simulink library "lib_FaultDetection"  (R2017a)
settings: Solver=VariableStepAuto  StartTime=0.0  StopTime=10.0  RelTol=1e-3
undefined symbols (not defined in the file): cal, ENGTRQ_MSMCH_Degraded_CP, ENGTRQ_MSMCH_ErrCritical_CP, ENGTRQ_MSMCH_LimpHome_CP
libraries: simulink x57, Diagnostic x4, lib_SystemDiag x1
(part 2 of 3)

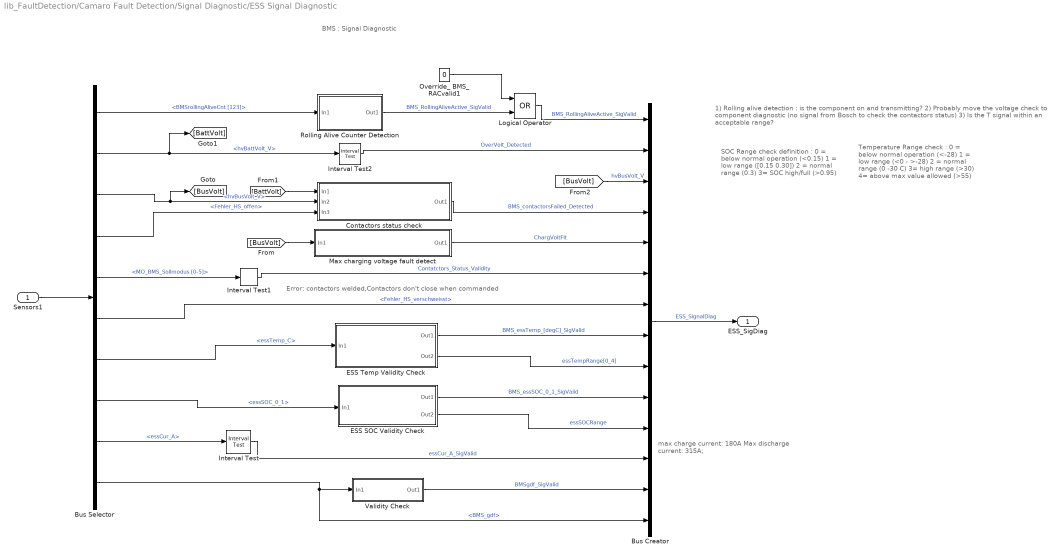
== system lib_FaultDetection/Camaro Fault Detection/Signal Diagnostic/ESS Signal Diagnostic ==
  note: BMS : Signal Diagnostic
  note: 1) Rolling alive detection : is the component on and transmitting?
      | 2) Probably move the voltage check to component diagnostic (no signal from Bosch to check the contactors status)
      | 3) Is  the T signal within an acceptable range?
  note: SOC Range check definition :
      | 0 = below normal operation (<0.15)
      | 1 = low range ([0.15 0.30])
      | 2 = normal range (0.3)
      | 3= SOC high/full (>0.95)
  note: Temperature Range check :
      | 0 = below normal operation (<-28)
      | 1 = low range (<0 - >-28)
      | 2 = normal range (0 -30 C)
      | 3= high range (>30)
      | 4= above max value allowed (>55)
  note: Error: contactors welded,Contactors don't close when commanded
  note: max charge current: 180A
      | Max discharge current: 315A;
  Sensors1 : Inport
  Bus Creator : BusCreator  Inputs=14
  Bus Selector : BusSelector  OutputSignals=BMS_Conv.BMSrollingAliveCnt [123],BMS_Conv.hvBattVolt_V,BMS_Conv.hvBusVolt_V,BMS_Conv.Fehler_HS_offen,BMS_Conv.MO_BMS_Sollmodus [0-5],BMS_Conv.Fehler_HS_verschweisst,BMS_Conv.essTemp_C,BMS_Conv.essSOC_0_1,BMS_Conv.essCur_A,BMS_Conv.BMS_gdf
  Contactors status check : Subsystem
  ESS SOC Validity Check : Subsystem
  ESS Temp Validity Check : Subsystem
  Interval Test : simulink/Logic and Bit Operations/Interval Test  IntervalClosedRight=on  uplimit=180  IntervalClosedLeft=on  lowlimit=-315  OutDataTypeStr=boolean
  Interval Test1 : simulink/Logic and Bit Operations/Interval Test  IntervalClosedRight=on  uplimit=7  IntervalClosedLeft=on  lowlimit=0  OutDataTypeStr=boolean
  Interval Test2 : simulink/Logic and Bit Operations/Interval Test  IntervalClosedRight=on  uplimit=430  IntervalClosedLeft=on  lowlimit=291  OutDataTypeStr=boolean
  Logical Operator : Logic  Operator=OR  AllPortsSameDT=off  OutDataTypeStr=boolean
  Max charging voltage fault detect : Subsystem
  Override_ BMS_RACvalid1 : Constant  Value=0
  Rolling Alive Counter Detection : Subsystem
  Validity Check : Subsystem
  ESS_SigDiag : Outport
  wires:
  Override_ BMS_RACvalid1/1 -> Logical Operator/1
  Rolling Alive Counter Detection/1(Out1) -> Logical Operator/2  "BMS_RollingAliveActive_SigValid"
  [BusVolt] -> Bus Creator/3  "hvBusVolt_V"
  Max charging voltage fault detect/1(Out1) -> Bus Creator/5  "ChargVoltFlt"
  [BusVolt] -> Max charging voltage fault detect/1(In1)
  [BattVolt] -> Contactors status check/1(In1)
  Interval Test2/1 -> Bus Creator/2  "OverVolt_Detected"
  Interval Test1/1 -> Bus Creator/6  "Contatctors_Status_Validity"
  Bus Selector/5 -> Interval Test1/1  "<MO_BMS_Sollmodus [0-5]>"
  Bus Selector/6 -> Bus Creator/7  "<Fehler_HS_verschweisst>"
  Contactors status check/1(Out1) -> Bus Creator/4  "BMS_contactorsFailed_Detected"
  Bus Selector/4 -> Contactors status check/3(In3)  "<Fehler_HS_offen>"
  Bus Selector/3 -> [BusVolt], Contactors status check/2(In2)  "<hvBusVolt_V>"
  ESS Temp Validity Check/2(Out2) -> Bus Creator/9  "essTempRange[0_4]"
  ESS Temp Validity Check/1(Out1) -> Bus Creator/8  "BMS_essTemp_[degC]_SigValid"
  Bus Selector/7 -> ESS Temp Validity Check/1(In1)  "<essTemp_C>"
  ESS SOC Validity Check/2(Out2) -> Bus Creator/11  "essSOCRange"
  ESS SOC Validity Check/1(Out1) -> Bus Creator/10  "BMS_essSOC_0_1_SigValid"
  Bus Selector/8 -> ESS SOC Validity Check/1(In1)  "<essSOC_0_1>"
  Validity Check/1(Out1) -> Bus Creator/13  "BMSgdf_SigValid"
  Bus Selector/10 -> Validity Check/1(In1), Bus Creator/14  "<BMS_gdf>"
  Interval Test/1 -> Bus Creator/12  "essCur_A_SigValid"
  Bus Selector/9 -> Interval Test/1  "<essCur_A>"
  Bus Creator/1 -> ESS_SigDiag/1  "ESS_SignalDiag"
  Bus Selector/2 -> [BattVolt], Interval Test2/1  "<hvBattVolt_V>"
  Logical Operator/1 -> Bus Creator/1  "BMS_RollingAliveActive_SigValid"
  Bus Selector/1 -> Rolling Alive Counter Detection/1(In1)  "<BMSrollingAliveCnt [123]>"
  Sensors1/1 -> Bus Selector/1

== system lib_FaultDetection/Camaro Fault Detection/Signal Diagnostic/Engine Signal Diagnostic ==
  note: Engine_Temp:
      | Normal range: <100
      | above max:>120
      | Limited range: 100-120
  note: ECM : Signal Diagnostic
  Sensors1 : Inport
  Bus Creator : BusCreator  Inputs=9
  Bus Selector : BusSelector  OutputSignals=ECM_Conv.ECMrollingAliveCnt [123],ECM_Conv.ECMTrqCmd_Nm,ECM_Conv.EngActStdyStTorq_Nm,ECM_Conv.EngineSpeed_rpm,ECM_Conv.Engine_Temp[DegC],ECM_Conv.EngRunAtv
  Constant1 : Constant
  Eng Feedback Trq Range Valid? : simulink/Logic and Bit Operations/Interval Test  IntervalClosedRight=on  uplimit=233  IntervalClosedLeft=on  lowlimit=0  OutDataTypeStr=boolean
  Eng Trq Range Valid? : simulink/Logic and Bit Operations/Interval Test  IntervalClosedRight=on  uplimit=233  IntervalClosedLeft=on  lowlimit=0  OutDataTypeStr=boolean
  EngTempValidity_Check : Subsystem
  Engine Run Active Valid? : simulink/Logic and Bit Operations/Interval Test  IntervalClosedRight=on  uplimit=1  IntervalClosedLeft=on  lowlimit=0  OutDataTypeStr=boolean
  Engine Speed Range Valid? : simulink/Logic and Bit Operations/Interval Test  IntervalClosedRight=on  uplimit=6500  IntervalClosedLeft=on  lowlimit=0  OutDataTypeStr=boolean
  Engine_Temp[DegC] : Stateflow chart  TreatAsAtomicUnit=on
  Rolling Alive Counter Detection1 : Subsystem
  Engine_SigDiag : Outport
  wires:
  EngTempValidity_Check/1(Out1) -> Bus Creator/7  "Eng_TempValid"
  Engine_Temp[DegC]/1(EngTempRange) -> Bus Creator/8, EngTempValidity_Check/1(In1)  "Eng_TempRange[123]"
  Constant1/1 -> Engine_Temp[DegC]/1(clearFaults)
  Engine Run Active Valid?/1 -> Bus Creator/9  "EngRunAtValid"
  Bus Selector/6 -> Engine Run Active Valid?/1  "<EngRunAtv>"
  Bus Selector/5 -> Engine_Temp[DegC]/2(Engine_Temp_DegC)  "<Engine_Temp[DegC]>"
  Eng Feedback Trq Range Valid?/1 -> Bus Creator/4  "EngActStdyStTorq_SigValid"
  Bus Selector/3 -> Eng Feedback Trq Range Valid?/1, Bus Creator/5  "<EngActStdyStTorq_Nm>"
  Engine Speed Range Valid?/1 -> Bus Creator/6  "Engine_Speed_rpm_SigValid"
  Bus Selector/4 -> Engine Speed Range Valid?/1  "<EngineSpeed_rpm>"
  Bus Creator/1 -> Engine_SigDiag/1  "Engine_SignalDiag"
  Eng Trq Range Valid?/1 -> Bus Creator/3  "engTrqCmdRecvd_SigValid"
  Bus Selector/2 -> Eng Trq Range Valid?/1, Bus Creator/2  "<ECMTrqCmd_Nm>"
  Rolling Alive Counter Detection1/1(Out1) -> Bus Creator/1  "ECMRollingAliveActive"
  Bus Selector/1 -> Rolling Alive Counter Detection1/1(In1)  "<ECMrollingAliveCnt [123]>"
  Sensors1/1 -> Bus Selector/1

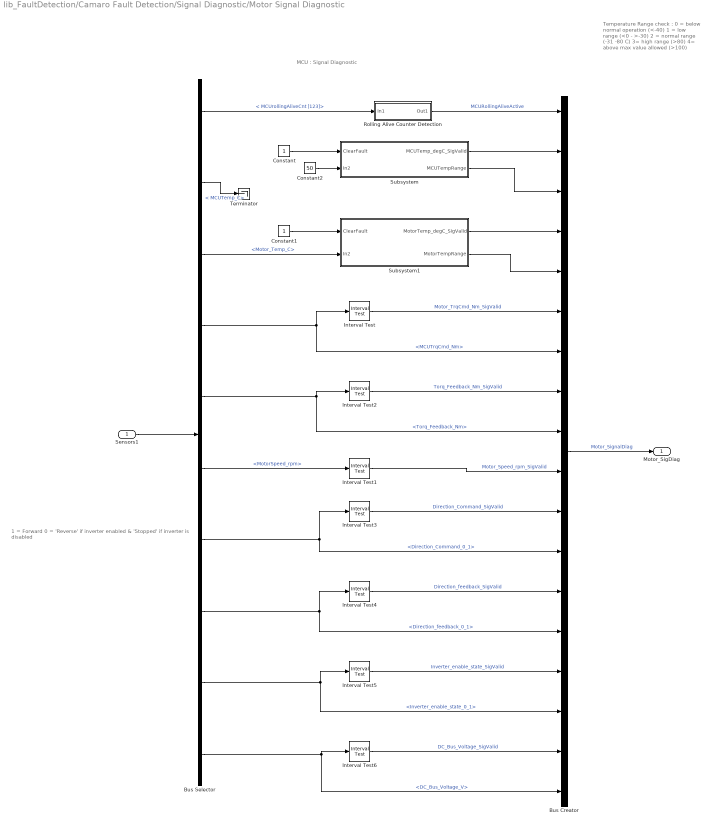
== system lib_FaultDetection/Camaro Fault Detection/Signal Diagnostic/Motor Signal Diagnostic ==
  note: 1 = Forward
      | 0 = 'Reverse' if inverter enabled  & 'Stopped' if inverter is disabled
  note: MCU : Signal Diagnostic
  note: Temperature Range check :
      | 0 = below normal operation (<-40)
      | 1 = low range (<0 - >-30)
      | 2 = normal range (-31 -80 C)
      | 3= high range (>80)
      | 4= above max value allowed (>100)
  Sensors1 : Inport
  Bus Creator : BusCreator  Inputs=18
  Bus Selector : BusSelector  OutputSignals=MCU_Conv.MCUrollingAliveCnt [123],MCU_Conv.MCUTemp_C,MCU_Conv.Motor_Temp_C,MCU_Conv.MCUTrqCmd_Nm,MCU_Conv.Torq_Feedback_Nm,MCU_Conv.MotorSpeed_rpm,MCU_Conv.Direction_Command_0_1,MCU_Conv.Direction_feedback_0_1,MCU_Conv.Inverter_enable_state_0_1,MCU_Conv.DC_Bus_Voltage_V
  Constant : Constant
  Constant1 : Constant
  Constant2 : Constant  Value=50
  Interval Test : simulink/Logic and Bit Operations/Interval Test  IntervalClosedRight=on  uplimit=350  IntervalClosedLeft=on  lowlimit=-350  OutDataTypeStr=boolean
  Interval Test1 : simulink/Logic and Bit Operations/Interval Test  IntervalClosedRight=on  uplimit=8000  IntervalClosedLeft=on  lowlimit=0  OutDataTypeStr=boolean
  Interval Test2 : simulink/Logic and Bit Operations/Interval Test  IntervalClosedRight=on  uplimit=350  IntervalClosedLeft=on  lowlimit=-350  OutDataTypeStr=boolean
  Interval Test3 : simulink/Logic and Bit Operations/Interval Test  IntervalClosedRight=on  uplimit=1  IntervalClosedLeft=on  lowlimit=0  OutDataTypeStr=boolean
  Interval Test4 : simulink/Logic and Bit Operations/Interval Test  IntervalClosedRight=on  uplimit=1  IntervalClosedLeft=on  lowlimit=0  OutDataTypeStr=boolean
  Interval Test5 : simulink/Logic and Bit Operations/Interval Test  IntervalClosedRight=on  uplimit=1  IntervalClosedLeft=on  lowlimit=0  OutDataTypeStr=boolean
  Interval Test6 : simulink/Logic and Bit Operations/Interval Test  IntervalClosedRight=on  uplimit=390  IntervalClosedLeft=on  lowlimit=-390  OutDataTypeStr=boolean
  Rolling Alive Counter Detection : Subsystem
  Subsystem : Subsystem
  Subsystem1 : Subsystem
  Terminator : Terminator
  Motor_SigDiag : Outport
  wires:
  Sensors1/1 -> Bus Selector/1
  Bus Selector/1 -> Rolling Alive Counter Detection/1(In1)  "< MCUrollingAliveCnt [123]>"
  Rolling Alive Counter Detection/1(Out1) -> Bus Creator/1  "MCURollingAliveActive"
  Bus Creator/1 -> Motor_SigDiag/1  "Motor_SignalDiag"
  Bus Selector/6 -> Interval Test1/1  "<MotorSpeed_rpm>"
  Interval Test1/1 -> Bus Creator/10  "Motor_Speed_rpm_SigValid"
  Interval Test/1 -> Bus Creator/6  "Motor_TrqCmd_Nm_SigValid"
  Bus Selector/4 -> Bus Creator/7, Interval Test/1  "<MCUTrqCmd_Nm>"
  Bus Selector/5 -> Interval Test2/1, Bus Creator/9  "<Torq_Feedback_Nm>"
  Interval Test2/1 -> Bus Creator/8  "Torq_Feedback_Nm_SigValid"
  Bus Selector/7 -> Interval Test3/1, Bus Creator/12  "<Direction_Command_0_1>"
  Interval Test3/1 -> Bus Creator/11  "Direction_Command_SigValid"
  Bus Selector/8 -> Interval Test4/1, Bus Creator/14  "<Direction_feedback_0_1>"
  Bus Selector/9 -> Interval Test5/1, Bus Creator/16  "<Inverter_enable_state_0_1>"
  Interval Test4/1 -> Bus Creator/13  "Direction_feedback_SigValid"
  Interval Test5/1 -> Bus Creator/15  "Inverter_enable_state_SigValid"
  Constant/1 -> Subsystem/1(ClearFault)
  Subsystem/1(MCUTemp_degC_SigValid) -> Bus Creator/2
  Constant1/1 -> Subsystem1/1(ClearFault)
  Bus Selector/3 -> Subsystem1/2(In2)  "<Motor_Temp_C>"
  Subsystem1/1(MotorTemp_degC_SigValid) -> Bus Creator/4
  Subsystem1/2(MotorTempRange) -> Bus Creator/5
  Bus Selector/10 -> Interval Test6/1, Bus Creator/18  "<DC_Bus_Voltage_V>"
  Interval Test6/1 -> Bus Creator/17  "DC_Bus_Voltage_SigValid"
  Subsystem/2(MCUTempRange) -> Bus Creator/3
  Bus Selector/2 -> Terminator/1  "< MCUTemp_C>"
  Constant2/1 -> Subsystem/2(In2)

== system lib_FaultDetection/Camaro Fault Detection/Signal Diagnostic/Subsystem1 ==
  note: Signal Naming Rule
      | Example: xxx_yyy_[z]_SigValid
      | xxx: source of the signal (Drv, Clu, BCM, ECM, TCM, BMS and MCU)
      | yyy: description of the signal
      | z: unit of the signal (V, A, Nm, m/s, %, 01, 0123, etc.)
  note: Signal Valid Setting Rule
      | xxx_yyy_[z]_SigValid could be 0 or 1
      | 0: signal invalid
      | 1: signal vaild

== system lib_FaultDetection/Camaro Fault Detection/Signal Diagnostic/Transmission Signal Diagnostic ==
  note: Lever Position:
      | 1 P
      | 2 R
      | 3 N
      | 4 D
      | 0: L
  note: TransEstGear
      | 0 : Not Supported
      | 1 : First Gear
      | 2 : Second Gear
      | 3 : Third Gear
      | 4 : Fourth Gear
      | 5 : Fifth Gear
      | 6 : Sixth Gear
      | 7 : Seventh Gear
      | 8 : Eight Gear
      | 10: EVT Mode 1
      | 11: EVT Mode 2
      | 12: CVT Forward Gear
      | 13: Neutral Gear
      | 14: Reverse Gear
      | 15: Park Gear
  note: TCM : Signal Diagnostic
  Sensors1 : Inport
  Bus Creator : BusCreator  Inputs=5
  Bus Selector : BusSelector  OutputSignals=TCM_Conv.CCMRollingAliveCnt [123],TCM_Conv.LvrPosTrnsShft,TCM_Conv.TransEstGear,DriverControls_Conv.V [mph],TCM_Conv.LockupCmd_0_1
  Interval Test : simulink/Logic and Bit Operations/Interval Test  IntervalClosedRight=on  uplimit=4  IntervalClosedLeft=on  lowlimit=0  OutDataTypeStr=boolean
  Interval Test1 : simulink/Logic and Bit Operations/Interval Test  IntervalClosedRight=on  uplimit=15  IntervalClosedLeft=on  lowlimit=0  OutDataTypeStr=boolean
  Interval Test2 : simulink/Logic and Bit Operations/Interval Test  IntervalClosedRight=on  uplimit=1  IntervalClosedLeft=on  lowlimit=0  OutDataTypeStr=boolean
  Rolling Alive Counter Detection : Subsystem
  Vehicle Direction Fault Detection : Subsystem
  Transmission_SigDiag : Outport
  wires:
  Vehicle Direction Fault Detection/1(Out1) -> Bus Creator/4  "VehDirFault"
  Interval Test2/1 -> Bus Creator/5  "LockupCmd_SigValid"
  Interval Test1/1 -> Bus Creator/3  "TransEstGear_SigValid"
  Interval Test/1 -> Bus Creator/2  "LvrPosTrnsShft_SigValid"
  Bus Selector/5 -> Interval Test2/1  "<LockupCmd_0_1>"
  Bus Selector/3 -> Interval Test1/1  "<TransEstGear>"
  Bus Selector/2 -> Interval Test/1, Vehicle Direction Fault Detection/1(LvrPosTrnsShft)  "<LvrPosTrnsShft>"
  Bus Creator/1 -> Transmission_SigDiag/1
  Rolling Alive Counter Detection/1(Out1) -> Bus Creator/1  "TCMRollingAliveActive_SigValid"
  Bus Selector/1 -> Rolling Alive Counter Detection/1(In1)  "<CCMRollingAliveCnt [123]>"
  Sensors1/1 -> Bus Selector/1
  Bus Selector/4 -> Vehicle Direction Fault Detection/2(Speed)  "<V [mph]>"

== system lib_FaultDetection/Camaro Fault Detection/Component Diagnostic/Engine Component Diagnostic/Override  engTrqCmd ==
  note: Override Switch Subsystem
  note: This subsystem is used to override the model value of a signal to a constant value
  In1 : Inport
  Constant : Constant  Value=50
  Multiport Switch : MultiPortSwitch  DataPortOrder=Zero-based contiguous  Inputs=2  zeroidx=on
  Signal Override Switch 0 = Use Model 1 = Use Constant : Constant
  Out1 : Outport
  wires:
  Constant/1 -> Multiport Switch/3
  Multiport Switch/1 -> Out1/1
  In1/1 -> Multiport Switch/2
  Signal Override Switch 0 = Use Model 1 = Use Constant/1 -> Multiport Switch/1

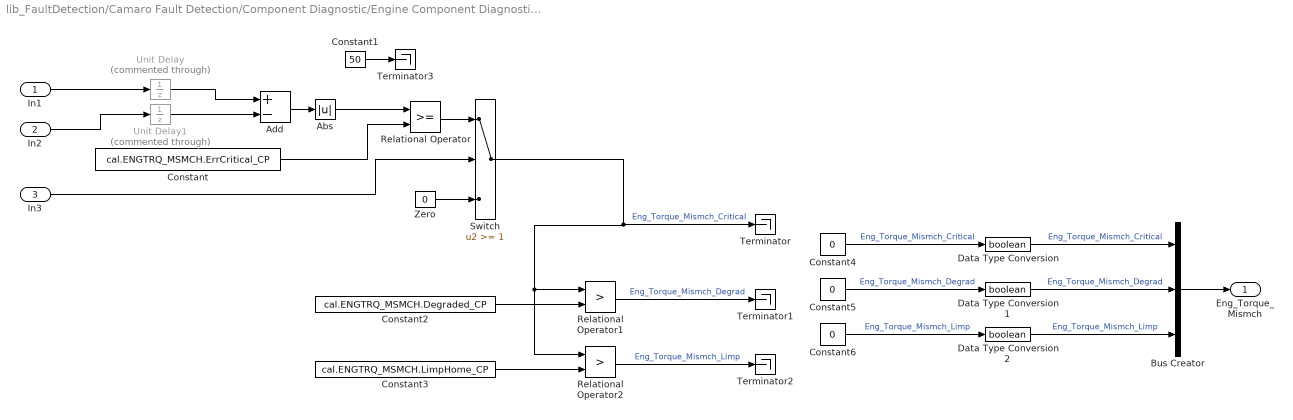
== system lib_FaultDetection/Camaro Fault Detection/Component Diagnostic/Engine Component Diagnostic/TorqMismatch Detection ==
  In1 : Inport
  In2 : Inport  Port=2
  In3 : Inport  Port=3
  Abs : Abs
  Add : Sum  Inputs=+-
  Bus Creator : BusCreator  Inputs=3
  Constant : Constant  Value=cal.ENGTRQ_MSMCH.ErrCritical_CP
  Constant1 : Constant  Value=50
  Constant2 : Constant  Value=cal.ENGTRQ_MSMCH.Degraded_CP
  Constant3 : Constant  Value=cal.ENGTRQ_MSMCH.LimpHome_CP
  Constant4 : Constant  Value=0
  Constant5 : Constant  Value=0
  Constant6 : Constant  Value=0
  Data Type Conversion : DataTypeConversion  OutDataTypeStr=boolean
  Data Type Conversion1 : DataTypeConversion  OutDataTypeStr=boolean
  Data Type Conversion2 : DataTypeConversion  OutDataTypeStr=boolean
  Relational Operator : RelationalOperator  OutDataTypeStr=boolean  RndMeth=Nearest
  Relational Operator1 : RelationalOperator  Operator=>  OutDataTypeStr=boolean  RndMeth=Nearest
  Relational Operator2 : RelationalOperator  Operator=>  OutDataTypeStr=boolean  RndMeth=Nearest
  Switch : Switch  Threshold=1
  Terminator{,1..3} (4 alike) : Terminator
  Unit Delay : UnitDelay  Commented=through  SampleTime=-1
  Unit Delay1 : UnitDelay  Commented=through  SampleTime=-1
  "Zero " : Constant  Value=0
  Eng_Torque_Mismch : Outport
  wires:
  Data Type Conversion2/1 -> Bus Creator/3  "Eng_Torque_Mismch_Limp"
  Data Type Conversion1/1 -> Bus Creator/2  "Eng_Torque_Mismch_Degrad"
  Data Type Conversion/1 -> Bus Creator/1  "Eng_Torque_Mismch_Critical"
  Constant5/1 -> Data Type Conversion1/1  "Eng_Torque_Mismch_Degrad"
  Constant6/1 -> Data Type Conversion2/1  "Eng_Torque_Mismch_Limp"
  Constant4/1 -> Data Type Conversion/1  "Eng_Torque_Mismch_Critical"
  Abs/1 -> Relational Operator/1
  Unit Delay1/1 -> Add/2
  Bus Creator/1 -> Eng_Torque_Mismch/1
  Relational Operator2/1 -> Terminator2/1  "Eng_Torque_Mismch_Limp"
  Relational Operator1/1 -> Terminator1/1  "Eng_Torque_Mismch_Degrad"
  Constant3/1 -> Relational Operator2/2
  Constant2/1 -> Relational Operator1/2
  Switch/1 -> Terminator/1, Relational Operator1/1, Relational Operator2/1  "Eng_Torque_Mismch_Critical"
  Relational Operator/1 -> Switch/1
  Add/1 -> Abs/1
  Constant/1 -> Relational Operator/2
  Unit Delay/1 -> Add/1
  In3/1 -> Switch/2
  "Zero "/1 -> Switch/3
  In2/1 -> Unit Delay1/1
  In1/1 -> Unit Delay/1
  Constant1/1 -> Terminator3/1

== system lib_FaultDetection/Camaro Fault Detection/Component Diagnostic/Motor Component Diagnostic/MCU_ESS_Voltage_Mismatch ==
  MCU_Voltage : Inport
  ESS_Voltage : Inport  Port=2
  Abs : Abs
  Add : Sum  Inputs=-+
  Constant : Constant  Value=cal.Diag.MCU.ESSVLT_MSMCH
  Relational Operator : RelationalOperator  OutDataTypeStr=boolean  RndMeth=Nearest
  MCU_ESS_Voltage_Mismch : Outport
  wires:
  Relational Operator/1 -> MCU_ESS_Voltage_Mismch/1
  Constant/1 -> Relational Operator/2
  Abs/1 -> Relational Operator/1
  ESS_Voltage/1 -> Add/2
  Add/1 -> Abs/1
  MCU_Voltage/1 -> Add/1

== system lib_FaultDetection/Camaro Fault Detection/Component Diagnostic/Motor Component Diagnostic/Motor_Direction_Mismatch ==
  note: 1: mismatch
      | 0: no failure
  Direction_Command : Inport
  Direction_Feedback : Inport  Port=2
  Inverter_enable_state : Inport  Port=3
  Logical Operator : Logic  AllPortsSameDT=off  OutDataTypeStr=boolean
  Relational Operator : RelationalOperator  Operator=~=  OutDataTypeStr=boolean  RndMeth=Nearest
  Direction_Mismch : Outport
  wires:
  Relational Operator/1 -> Logical Operator/1
  Logical Operator/1 -> Direction_Mismch/1
  Direction_Command/1 -> Relational Operator/1  "Direction_Command"
  Direction_Feedback/1 -> Relational Operator/2  "Direction_Feedback"
  Inverter_enable_state/1 -> Logical Operator/2  "Inverter_enable_state"

== system lib_FaultDetection/Camaro Fault Detection/Component Diagnostic/Motor Component Diagnostic/Override  fault ==
  note: This subsystem is used to override the model value of a signal to a constant value
  note: Override Switch Subsystem
  In1 : Inport
  Multiport Switch : MultiPortSwitch  DataPortOrder=Zero-based contiguous  Inputs=2  zeroidx=on
  Override Value : Constant  Value=0  OutDataTypeStr=double
  Signal Override Switch 0 = Use Model 1 = Use Constant : Constant
  Out1 : Outport
  wires:
  Signal Override Switch 0 = Use Model 1 = Use Constant/1 -> Multiport Switch/1
  In1/1 -> Multiport Switch/2
  Multiport Switch/1 -> Out1/1
  Override Value/1 -> Multiport Switch/3

== system lib_FaultDetection/Camaro Fault Detection/Component Diagnostic/Motor Component Diagnostic/Override  fault1 ==
  note: Override Switch Subsystem
  note: This subsystem is used to override the model value of a signal to a constant value
  In1 : Inport
  Multiport Switch : MultiPortSwitch  DataPortOrder=Zero-based contiguous  Inputs=2  zeroidx=on
  Override Value : Constant  Value=0  OutDataTypeStr=double
  Signal Override Switch 0 = Use Model 1 = Use Constant : Constant  Value=0
  Out1 : Outport
  wires:
  Override Value/1 -> Multiport Switch/3
  Multiport Switch/1 -> Out1/1
  In1/1 -> Multiport Switch/2
  Signal Override Switch 0 = Use Model 1 = Use Constant/1 -> Multiport Switch/1

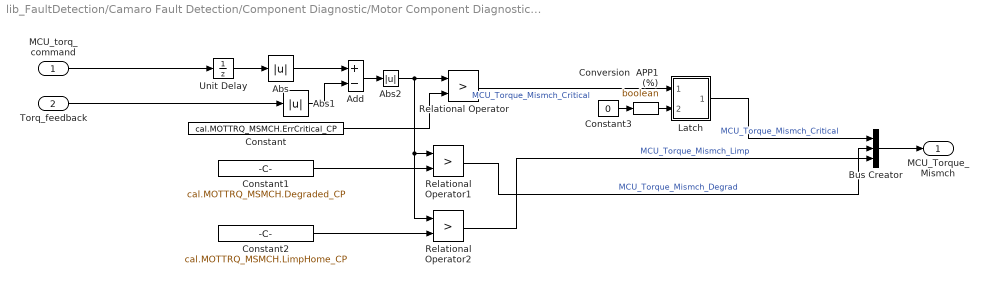
== system lib_FaultDetection/Camaro Fault Detection/Component Diagnostic/Motor Component Diagnostic/Torque_Mismatch ==
  MCU_torq_command : Inport
  Torq_feedback : Inport  Port=2
  Abs : Abs
  Abs1 : Abs
  Abs2 : Abs
  Add : Sum  Inputs=+-
  Bus Creator : BusCreator  Inputs=3
  Constant : Constant  Value=cal.MOTTRQ_MSMCH.ErrCritical_CP
  Constant1 : Constant  Value=cal.MOTTRQ_MSMCH.Degraded_CP
  Constant2 : Constant  Value=cal.MOTTRQ_MSMCH.LimpHome_CP
  Constant3 : Constant  Value=0
  Conversion  APP1 (%) : DataTypeConversion  OutDataTypeStr=boolean
  Latch : Subsystem
  Relational Operator : RelationalOperator  Operator=>  OutDataTypeStr=boolean  RndMeth=Nearest
  Relational Operator1 : RelationalOperator  Operator=>  OutDataTypeStr=boolean  RndMeth=Nearest
  Relational Operator2 : RelationalOperator  Operator=>  OutDataTypeStr=boolean  RndMeth=Nearest
  Unit Delay : UnitDelay  SampleTime=-1
  MCU_Torque_Mismch : Outport
  wires:
  Unit Delay/1 -> Abs/1
  Abs/1 -> Add/1
  Torq_feedback/1 -> Abs1/1
  Abs1/1 -> Add/2
  MCU_torq_command/1 -> Unit Delay/1
  Constant/1 -> Relational Operator/2
  Constant1/1 -> Relational Operator1/2
  Constant2/1 -> Relational Operator2/2
  Relational Operator1/1 -> Bus Creator/2  "MCU_Torque_Mismch_Degrad"
  Relational Operator2/1 -> Bus Creator/3  "MCU_Torque_Mismch_Limp"
  Bus Creator/1 -> MCU_Torque_Mismch/1
  Add/1 -> Abs2/1
  Abs2/1 -> Relational Operator/1, Relational Operator2/1, Relational Operator1/1
  Constant3/1 -> Conversion  APP1 (%)/1
  Relational Operator/1 -> Latch/1(In1)  "MCU_Torque_Mismch_Critical"
  Latch/1(Out1) -> Bus Creator/1  "MCU_Torque_Mismch_Critical"
  Conversion  APP1 (%)/1 -> Latch/2(In2)

== system lib_FaultDetection/Camaro Fault Detection/Input Conversions/BMS_Conversions/Override  BMS_gdf 0_1 ==
  note: This subsystem is used to override the model value of a signal to a constant value
  note: Override Switch Subsystem
  In1 : Inport
  Multiport Switch : MultiPortSwitch  DataPortOrder=Zero-based contiguous  Inputs=2  zeroidx=on
  Override Value : Constant  Value=0  OutDataTypeStr=double
  Signal Override Switch 0 = Use Model 1 = Use Constant : Constant
  Out1 : Outport
  wires:
  Signal Override Switch 0 = Use Model 1 = Use Constant/1 -> Multiport Switch/1
  In1/1 -> Multiport Switch/2
  Multiport Switch/1 -> Out1/1
  Override Value/1 -> Multiport Switch/3

== system lib_FaultDetection/Camaro Fault Detection/Input Conversions/BMS_Conversions/Override  closeContactorsCmd ==
  note: Override Switch Subsystem
  note: This subsystem is used to override the model value of a signal to a constant value
  In1 : Inport
  Multiport Switch : MultiPortSwitch  DataPortOrder=Zero-based contiguous  Inputs=2  zeroidx=on
  Override Value : Constant  Value=0  OutDataTypeStr=double
  Signal Override Switch 0 = Use Model 1 = Use Constant : Constant  Value=0
  Out1 : Outport
  wires:
  Override Value/1 -> Multiport Switch/3
  Multiport Switch/1 -> Out1/1
  In1/1 -> Multiport Switch/2
  Signal Override Switch 0 = Use Model 1 = Use Constant/1 -> Multiport Switch/1

== system lib_FaultDetection/Camaro Fault Detection/Input Conversions/BMS_Conversions/Override  contactorsClsd ==
  note: Override Switch Subsystem
  note: This subsystem is used to override the model value of a signal to a constant value
  In1 : Inport
  Multiport Switch : MultiPortSwitch  DataPortOrder=Zero-based contiguous  Inputs=2  zeroidx=on
  Override Value : Constant  Value=0  OutDataTypeStr=double
  Signal Override Switch 0 = Use Model 1 = Use Constant : Constant  Value=0
  Out1 : Outport
  wires:
  Override Value/1 -> Multiport Switch/3
  Multiport Switch/1 -> Out1/1
  In1/1 -> Multiport Switch/2
  Signal Override Switch 0 = Use Model 1 = Use Constant/1 -> Multiport Switch/1

== system lib_FaultDetection/Camaro Fault Detection/Input Conversions/BMS_Conversions/Override  essCur_A ==
  note: This subsystem is used to override the model value of a signal to a constant value
  note: Override Switch Subsystem
  In1 : Inport
  Multiport Switch : MultiPortSwitch  DataPortOrder=Zero-based contiguous  Inputs=2  zeroidx=on
  Override Value : Constant  Value=0  OutDataTypeStr=double
  Signal Override Switch 0 = Use Model 1 = Use Constant : Constant  Value=0
  Out1 : Outport
  wires:
  Signal Override Switch 0 = Use Model 1 = Use Constant/1 -> Multiport Switch/1
  In1/1 -> Multiport Switch/2
  Multiport Switch/1 -> Out1/1
  Override Value/1 -> Multiport Switch/3

== system lib_FaultDetection/Camaro Fault Detection/Input Conversions/BMS_Conversions/Override  essSOC_0_1 ==
  note: Override Switch Subsystem
  note: This subsystem is used to override the model value of a signal to a constant value
  In1 : Inport
  Multiport Switch : MultiPortSwitch  DataPortOrder=Zero-based contiguous  Inputs=2  zeroidx=on
  Override Value : Constant  Value=0  OutDataTypeStr=double
  Signal Override Switch 0 = Use Model 1 = Use Constant : Constant  Value=0
  Out1 : Outport
  wires:
  Override Value/1 -> Multiport Switch/3
  Multiport Switch/1 -> Out1/1
  In1/1 -> Multiport Switch/2
  Signal Override Switch 0 = Use Model 1 = Use Constant/1 -> Multiport Switch/1

== system lib_FaultDetection/Camaro Fault Detection/Input Conversions/BMS_Conversions/Override  essTemp_C ==
  note: Override Switch Subsystem
  note: This subsystem is used to override the model value of a signal to a constant value
  In1 : Inport
  Multiport Switch : MultiPortSwitch  DataPortOrder=Zero-based contiguous  Inputs=2  zeroidx=on
  Override Value : Constant  Value=0  OutDataTypeStr=double
  Signal Override Switch 0 = Use Model 1 = Use Constant : Constant
  Out1 : Outport
  wires:
  Override Value/1 -> Multiport Switch/3
  Multiport Switch/1 -> Out1/1
  In1/1 -> Multiport Switch/2
  Signal Override Switch 0 = Use Model 1 = Use Constant/1 -> Multiport Switch/1

== system lib_FaultDetection/Camaro Fault Detection/Input Conversions/BMS_Conversions/Override  hvBattVolt_V ==
  note: Override Switch Subsystem
  note: This subsystem is used to override the model value of a signal to a constant value
  In1 : Inport
  Multiport Switch : MultiPortSwitch  DataPortOrder=Zero-based contiguous  Inputs=2  zeroidx=on
  Override Value : Constant  Value=0  OutDataTypeStr=double
  Signal Override Switch 0 = Use Model 1 = Use Constant : Constant  Value=0
  Out1 : Outport
  wires:
  Override Value/1 -> Multiport Switch/3
  Multiport Switch/1 -> Out1/1
  In1/1 -> Multiport Switch/2
  Signal Override Switch 0 = Use Model 1 = Use Constant/1 -> Multiport Switch/1

== system lib_FaultDetection/Camaro Fault Detection/Input Conversions/BMS_Conversions/Override  hvBusVolt_V ==
  note: This subsystem is used to override the model value of a signal to a constant value
  note: Override Switch Subsystem
  In1 : Inport
  Multiport Switch : MultiPortSwitch  DataPortOrder=Zero-based contiguous  Inputs=2  zeroidx=on
  Override Value : Constant  Value=0  OutDataTypeStr=double
  Signal Override Switch 0 = Use Model 1 = Use Constant : Constant  Value=0
  Out1 : Outport
  wires:
  Signal Override Switch 0 = Use Model 1 = Use Constant/1 -> Multiport Switch/1
  In1/1 -> Multiport Switch/2
  Multiport Switch/1 -> Out1/1
  Override Value/1 -> Multiport Switch/3

== system lib_FaultDetection/Camaro Fault Detection/Input Conversions/BMS_Conversions/Override  rollingAliveCnt [1_3] ==
  note: This subsystem is used to override the model value of a signal to a constant value
  note: Override Switch Subsystem
  In1 : Inport
  Multiport Switch : MultiPortSwitch  DataPortOrder=Zero-based contiguous  Inputs=2  zeroidx=on
  Override Value : Constant  Value=0  OutDataTypeStr=double
  Signal Override Switch 0 = Use Model 1 = Use Constant : Constant  Value=0
  Out1 : Outport
  wires:
  Signal Override Switch 0 = Use Model 1 = Use Constant/1 -> Multiport Switch/1
  In1/1 -> Multiport Switch/2
  Multiport Switch/1 -> Out1/1
  Override Value/1 -> Multiport Switch/3

== system lib_FaultDetection/Camaro Fault Detection/Input Conversions/BMS_Conversions/Override Fehler_HS_offen ==
  note: Override Switch Subsystem
  note: This subsystem is used to override the model value of a signal to a constant value
  In1 : Inport
  Multiport Switch : MultiPortSwitch  DataPortOrder=Zero-based contiguous  Inputs=2  zeroidx=on
  Override Value : Constant  Value=0  OutDataTypeStr=double
  Signal Override Switch 0 = Use Model 1 = Use Constant : Constant
  Out1 : Outport
  wires:
  Override Value/1 -> Multiport Switch/3
  Multiport Switch/1 -> Out1/1
  In1/1 -> Multiport Switch/2
  Signal Override Switch 0 = Use Model 1 = Use Constant/1 -> Multiport Switch/1

== system lib_FaultDetection/Camaro Fault Detection/Input Conversions/BMS_Conversions/Override Fehler_HS_verschweisst ==
  note: This subsystem is used to override the model value of a signal to a constant value
  note: Override Switch Subsystem
  In1 : Inport
  Multiport Switch : MultiPortSwitch  DataPortOrder=Zero-based contiguous  Inputs=2  zeroidx=on
  Override Value : Constant  Value=0  OutDataTypeStr=double
  Signal Override Switch 0 = Use Model 1 = Use Constant : Constant
  Out1 : Outport
  wires:
  Signal Override Switch 0 = Use Model 1 = Use Constant/1 -> Multiport Switch/1
  In1/1 -> Multiport Switch/2
  Multiport Switch/1 -> Out1/1
  Override Value/1 -> Multiport Switch/3

== system lib_FaultDetection/Camaro Fault Detection/Input Conversions/Clutch_Conversions/Override  rollingAliveCnt [123] ==
  note: This subsystem is used to override the model value of a signal to a constant value
  note: Override Switch Subsystem
  In1 : Inport
  Multiport Switch : MultiPortSwitch  DataPortOrder=Zero-based contiguous  Inputs=2  zeroidx=on
  Override Value : Constant  Value=0  OutDataTypeStr=double
  Signal Override Switch 0 = Use Model 1 = Use Constant : Constant  Value=0
  Out1 : Outport
  wires:
  Signal Override Switch 0 = Use Model 1 = Use Constant/1 -> Multiport Switch/1
  In1/1 -> Multiport Switch/2
  Multiport Switch/1 -> Out1/1
  Override Value/1 -> Multiport Switch/3

== system lib_FaultDetection/Camaro Fault Detection/Input Conversions/Clutch_Conversions/Override Checksum [0-255] ==
  note: Override Switch Subsystem
  note: This subsystem is used to override the model value of a signal to a constant value
  In1 : Inport
  Multiport Switch : MultiPortSwitch  DataPortOrder=Zero-based contiguous  Inputs=2  zeroidx=on
  Override Value : Constant  Value=0  OutDataTypeStr=double
  Signal Override Switch 0 = Use Model 1 = Use Constant : Constant  Value=0
  Out1 : Outport
  wires:
  Override Value/1 -> Multiport Switch/3
  Multiport Switch/1 -> Out1/1
  In1/1 -> Multiport Switch/2
  Signal Override Switch 0 = Use Model 1 = Use Constant/1 -> Multiport Switch/1

== system lib_FaultDetection/Camaro Fault Detection/Input Conversions/Clutch_Conversions/Override Error CAN [0-1] ==
  note: This subsystem is used to override the model value of a signal to a constant value
  note: Override Switch Subsystem
  In1 : Inport
  Multiport Switch : MultiPortSwitch  DataPortOrder=Zero-based contiguous  Inputs=2  zeroidx=on
  Override Value : Constant  Value=0  OutDataTypeStr=double
  Signal Override Switch 0 = Use Model 1 = Use Constant : Constant  Value=0
  Out1 : Outport
  wires:
  Signal Override Switch 0 = Use Model 1 = Use Constant/1 -> Multiport Switch/1
  In1/1 -> Multiport Switch/2
  Multiport Switch/1 -> Out1/1
  Override Value/1 -> Multiport Switch/3

== system lib_FaultDetection/Camaro Fault Detection/Input Conversions/Clutch_Conversions/Override Error Hardware [0-1] ==
  note: Override Switch Subsystem
  note: This subsystem is used to override the model value of a signal to a constant value
  In1 : Inport
  Multiport Switch : MultiPortSwitch  DataPortOrder=Zero-based contiguous  Inputs=2  zeroidx=on
  Override Value : Constant  Value=0  OutDataTypeStr=double
  Signal Override Switch 0 = Use Model 1 = Use Constant : Constant  Value=0
  Out1 : Outport
  wires:
  Override Value/1 -> Multiport Switch/3
  Multiport Switch/1 -> Out1/1
  In1/1 -> Multiport Switch/2
  Signal Override Switch 0 = Use Model 1 = Use Constant/1 -> Multiport Switch/1

== system lib_FaultDetection/Camaro Fault Detection/Input Conversions/Clutch_Conversions/Override Error Mechanical [0-1] ==
  note: This subsystem is used to override the model value of a signal to a constant value
  note: Override Switch Subsystem
  In1 : Inport
  Multiport Switch : MultiPortSwitch  DataPortOrder=Zero-based contiguous  Inputs=2  zeroidx=on
  Override Value : Constant  Value=0  OutDataTypeStr=double
  Signal Override Switch 0 = Use Model 1 = Use Constant : Constant  Value=0
  Out1 : Outport
  wires:
  Signal Override Switch 0 = Use Model 1 = Use Constant/1 -> Multiport Switch/1
  In1/1 -> Multiport Switch/2
  Multiport Switch/1 -> Out1/1
  Override Value/1 -> Multiport Switch/3

== system lib_FaultDetection/Camaro Fault Detection/Input Conversions/Clutch_Conversions/Override Mode [0-7] ==
  note: This subsystem is used to override the model value of a signal to a constant value
  note: Override Switch Subsystem
  In1 : Inport
  Multiport Switch : MultiPortSwitch  DataPortOrder=Zero-based contiguous  Inputs=2  zeroidx=on
  Override Value : Constant  Value=0  OutDataTypeStr=double
  Signal Override Switch 0 = Use Model 1 = Use Constant : Constant  Value=0
  Out1 : Outport
  wires:
  Signal Override Switch 0 = Use Model 1 = Use Constant/1 -> Multiport Switch/1
  In1/1 -> Multiport Switch/2
  Multiport Switch/1 -> Out1/1
  Override Value/1 -> Multiport Switch/3

== system lib_FaultDetection/Camaro Fault Detection/Input Conversions/Clutch_Conversions/Override Position [deg] ==
  note: Override Switch Subsystem
  note: This subsystem is used to override the model value of a signal to a constant value
  In1 : Inport
  Multiport Switch : MultiPortSwitch  DataPortOrder=Zero-based contiguous  Inputs=2  zeroidx=on
  Override Value : Constant  Value=0  OutDataTypeStr=double
  Signal Override Switch 0 = Use Model 1 = Use Constant : Constant  Value=0
  Out1 : Outport
  wires:
  Override Value/1 -> Multiport Switch/3
  Multiport Switch/1 -> Out1/1
  In1/1 -> Multiport Switch/2
  Signal Override Switch 0 = Use Model 1 = Use Constant/1 -> Multiport Switch/1

== system lib_FaultDetection/Camaro Fault Detection/Input Conversions/Clutch_Conversions/Override Pressure [bar] ==
  note: This subsystem is used to override the model value of a signal to a constant value
  note: Override Switch Subsystem
  In1 : Inport
  Multiport Switch : MultiPortSwitch  DataPortOrder=Zero-based contiguous  Inputs=2  zeroidx=on
  Override Value : Constant  Value=0  OutDataTypeStr=double
  Signal Override Switch 0 = Use Model 1 = Use Constant : Constant  Value=0
  Out1 : Outport
  wires:
  Signal Override Switch 0 = Use Model 1 = Use Constant/1 -> Multiport Switch/1
  In1/1 -> Multiport Switch/2
  Multiport Switch/1 -> Out1/1
  Override Value/1 -> Multiport Switch/3

== system lib_FaultDetection/Camaro Fault Detection/Input Conversions/Clutch_Conversions/Override Temp Error [0-1] ==
  note: This subsystem is used to override the model value of a signal to a constant value
  note: Override Switch Subsystem
  In1 : Inport
  Multiport Switch : MultiPortSwitch  DataPortOrder=Zero-based contiguous  Inputs=2  zeroidx=on
  Override Value : Constant  Value=0  OutDataTypeStr=double
  Signal Override Switch 0 = Use Model 1 = Use Constant : Constant  Value=0
  Out1 : Outport
  wires:
  Signal Override Switch 0 = Use Model 1 = Use Constant/1 -> Multiport Switch/1
  In1/1 -> Multiport Switch/2
  Multiport Switch/1 -> Out1/1
  Override Value/1 -> Multiport Switch/3

== system lib_FaultDetection/Camaro Fault Detection/Input Conversions/Clutch_Conversions/Override Temp Warning [0-1] ==
  note: Override Switch Subsystem
  note: This subsystem is used to override the model value of a signal to a constant value
  In1 : Inport
  Multiport Switch : MultiPortSwitch  DataPortOrder=Zero-based contiguous  Inputs=2  zeroidx=on
  Override Value : Constant  Value=0  OutDataTypeStr=double
  Signal Override Switch 0 = Use Model 1 = Use Constant : Constant  Value=0
  Out1 : Outport
  wires:
  Override Value/1 -> Multiport Switch/3
  Multiport Switch/1 -> Out1/1
  In1/1 -> Multiport Switch/2
  Signal Override Switch 0 = Use Model 1 = Use Constant/1 -> Multiport Switch/1

== system lib_FaultDetection/Camaro Fault Detection/Input Conversions/Clutch_Conversions/Override Voltage Error [0-1] ==
  note: Override Switch Subsystem
  note: This subsystem is used to override the model value of a signal to a constant value
  In1 : Inport
  Multiport Switch : MultiPortSwitch  DataPortOrder=Zero-based contiguous  Inputs=2  zeroidx=on
  Override Value : Constant  Value=0  OutDataTypeStr=double
  Signal Override Switch 0 = Use Model 1 = Use Constant : Constant  Value=0
  Out1 : Outport
  wires:
  Override Value/1 -> Multiport Switch/3
  Multiport Switch/1 -> Out1/1
  In1/1 -> Multiport Switch/2
  Signal Override Switch 0 = Use Model 1 = Use Constant/1 -> Multiport Switch/1

== system lib_FaultDetection/Camaro Fault Detection/Input Conversions/DriverInput_Conversions/Override  KeyPos [0_3] ==
  note: This subsystem is used to override the model value of a signal to a constant value
  note: Override Switch Subsystem
  In1 : Inport
  Multiport Switch : MultiPortSwitch  DataPortOrder=Zero-based contiguous  Inputs=2  zeroidx=on
  Override Value : Constant  Value=0  OutDataTypeStr=double
  Signal Override Switch 0 = Use Model 1 = Use Constant : Constant  Value=0
  Out1 : Outport
  wires:
  Signal Override Switch 0 = Use Model 1 = Use Constant/1 -> Multiport Switch/1
  In1/1 -> Multiport Switch/2
  Multiport Switch/1 -> Out1/1
  Override Value/1 -> Multiport Switch/3

== system lib_FaultDetection/Camaro Fault Detection/Input Conversions/DriverInput_Conversions/Override APP (%) ==
  note: This subsystem is used to override the model value of a signal to a constant value
  note: Override Switch Subsystem
  In1 : Inport
  Multiport Switch : MultiPortSwitch  DataPortOrder=Zero-based contiguous  Inputs=2  zeroidx=on
  Override Value : Constant  Value=0  OutDataTypeStr=double
  Signal Override Switch 0 = Use Model 1 = Use Constant : Constant  Value=0
  Out1 : Outport
  wires:
  Signal Override Switch 0 = Use Model 1 = Use Constant/1 -> Multiport Switch/1
  In1/1 -> Multiport Switch/2
  Multiport Switch/1 -> Out1/1
  Override Value/1 -> Multiport Switch/3

== system lib_FaultDetection/Camaro Fault Detection/Input Conversions/DriverInput_Conversions/Override APP (%)1 ==
  note: Override Switch Subsystem
  note: This subsystem is used to override the model value of a signal to a constant value
  In1 : Inport
  Multiport Switch : MultiPortSwitch  DataPortOrder=Zero-based contiguous  Inputs=2  zeroidx=on
  Override Value : Constant  Value=0  OutDataTypeStr=double
  Signal Override Switch 0 = Use Model 1 = Use Constant : Constant  Value=0
  Out1 : Outport
  wires:
  Override Value/1 -> Multiport Switch/3
  Multiport Switch/1 -> Out1/1
  In1/1 -> Multiport Switch/2
  Signal Override Switch 0 = Use Model 1 = Use Constant/1 -> Multiport Switch/1

== system lib_FaultDetection/Camaro Fault Detection/Input Conversions/DriverInput_Conversions/Override BPP (%) ==
  note: Override Switch Subsystem
  note: This subsystem is used to override the model value of a signal to a constant value
  In1 : Inport
  Multiport Switch : MultiPortSwitch  DataPortOrder=Zero-based contiguous  Inputs=2  zeroidx=on
  Override Value : Constant  Value=0  OutDataTypeStr=double
  Signal Override Switch 0 = Use Model 1 = Use Constant : Constant  Value=0
  Out1 : Outport
  wires:
  Override Value/1 -> Multiport Switch/3
  Multiport Switch/1 -> Out1/1
  In1/1 -> Multiport Switch/2
  Signal Override Switch 0 = Use Model 1 = Use Constant/1 -> Multiport Switch/1

== system lib_FaultDetection/Camaro Fault Detection/Input Conversions/DriverInput_Conversions/Override PRNDL ==
  note: This subsystem is used to override the model value of a signal to a constant value
  note: Override Switch Subsystem
  In1 : Inport
  Multiport Switch : MultiPortSwitch  DataPortOrder=Zero-based contiguous  Inputs=2  zeroidx=on
  Override Value : Constant  Value=0  OutDataTypeStr=double
  Signal Override Switch 0 = Use Model 1 = Use Constant : Constant  Value=0
  Out1 : Outport
  wires:
  Signal Override Switch 0 = Use Model 1 = Use Constant/1 -> Multiport Switch/1
  In1/1 -> Multiport Switch/2
  Multiport Switch/1 -> Out1/1
  Override Value/1 -> Multiport Switch/3

== system lib_FaultDetection/Camaro Fault Detection/Input Conversions/DriverInput_Conversions/Override Regen ==
  note: This subsystem is used to override the model value of a signal to a constant value
  note: Override Switch Subsystem
  In1 : Inport
  Multiport Switch : MultiPortSwitch  DataPortOrder=Zero-based contiguous  Inputs=2  zeroidx=on
  Override Value : Constant  Value=0  OutDataTypeStr=double
  Signal Override Switch 0 = Use Model 1 = Use Constant : Constant  Value=0
  Out1 : Outport
  wires:
  Signal Override Switch 0 = Use Model 1 = Use Constant/1 -> Multiport Switch/1
  In1/1 -> Multiport Switch/2
  Multiport Switch/1 -> Out1/1
  Override Value/1 -> Multiport Switch/3

== system lib_FaultDetection/Camaro Fault Detection/Input Conversions/DriverInput_Conversions/Override V [mph] ==
  note: Override Switch Subsystem
  note: This subsystem is used to override the model value of a signal to a constant value
  In1 : Inport
  Multiport Switch : MultiPortSwitch  DataPortOrder=Zero-based contiguous  Inputs=2  zeroidx=on
  Override Value : Constant  Value=0  OutDataTypeStr=double
  Signal Override Switch 0 = Use Model 1 = Use Constant : Constant  Value=0
  Out1 : Outport
  wires:
  Override Value/1 -> Multiport Switch/3
  Multiport Switch/1 -> Out1/1
  In1/1 -> Multiport Switch/2
  Signal Override Switch 0 = Use Model 1 = Use Constant/1 -> Multiport Switch/1

== system lib_FaultDetection/Camaro Fault Detection/Input Conversions/ECM_Conversions/Override  ECMTrqCmd_Nm ==
  note: Override Switch Subsystem
  note: This subsystem is used to override the model value of a signal to a constant value
  In1 : Inport
  Multiport Switch : MultiPortSwitch  DataPortOrder=Zero-based contiguous  Inputs=2  zeroidx=on
  Override Value : Constant  Value=0  OutDataTypeStr=double
  Signal Override Switch 0 = Use Model 1 = Use Constant : Constant  Value=0
  Out1 : Outport
  wires:
  Override Value/1 -> Multiport Switch/3
  Multiport Switch/1 -> Out1/1
  In1/1 -> Multiport Switch/2
  Signal Override Switch 0 = Use Model 1 = Use Constant/1 -> Multiport Switch/1

== system lib_FaultDetection/Camaro Fault Detection/Input Conversions/ECM_Conversions/Override  ECMrollingAliveCnt ==
  note: This subsystem is used to override the model value of a signal to a constant value
  note: Override Switch Subsystem
  In1 : Inport
  Multiport Switch : MultiPortSwitch  DataPortOrder=Zero-based contiguous  Inputs=2  zeroidx=on
  Override Value : Constant  Value=0  OutDataTypeStr=double
  Signal Override Switch 0 = Use Model 1 = Use Constant : Constant  Value=0
  Out1 : Outport
  wires:
  Signal Override Switch 0 = Use Model 1 = Use Constant/1 -> Multiport Switch/1
  In1/1 -> Multiport Switch/2
  Multiport Switch/1 -> Out1/1
  Override Value/1 -> Multiport Switch/3

== system lib_FaultDetection/Camaro Fault Detection/Input Conversions/ECM_Conversions/Override  EngActStdyStTorq_Nm ==
  note: This subsystem is used to override the model value of a signal to a constant value
  note: Override Switch Subsystem
  In1 : Inport
  Multiport Switch : MultiPortSwitch  DataPortOrder=Zero-based contiguous  Inputs=2  zeroidx=on
  Override Value : Constant  Value=0  OutDataTypeStr=double
  Signal Override Switch 0 = Use Model 1 = Use Constant : Constant  Value=0
  Out1 : Outport
  wires:
  Signal Override Switch 0 = Use Model 1 = Use Constant/1 -> Multiport Switch/1
  In1/1 -> Multiport Switch/2
  Multiport Switch/1 -> Out1/1
  Override Value/1 -> Multiport Switch/3

== system lib_FaultDetection/Camaro Fault Detection/Input Conversions/ECM_Conversions/Override  EngRunAtv ==
  note: Override Switch Subsystem
  note: This subsystem is used to override the model value of a signal to a constant value
  In1 : Inport
  Multiport Switch : MultiPortSwitch  DataPortOrder=Zero-based contiguous  Inputs=2  zeroidx=on
  Override Value : Constant  Value=0  OutDataTypeStr=double
  Signal Override Switch 0 = Use Model 1 = Use Constant : Constant  Value=0
  Out1 : Outport
  wires:
  Override Value/1 -> Multiport Switch/3
  Multiport Switch/1 -> Out1/1
  In1/1 -> Multiport Switch/2
  Signal Override Switch 0 = Use Model 1 = Use Constant/1 -> Multiport Switch/1

== system lib_FaultDetection/Camaro Fault Detection/Input Conversions/ECM_Conversions/Override  EngineSpeed_rpm ==
  note: Override Switch Subsystem
  note: This subsystem is used to override the model value of a signal to a constant value
  In1 : Inport
  Multiport Switch : MultiPortSwitch  DataPortOrder=Zero-based contiguous  Inputs=2  zeroidx=on
  Override Value : Constant  Value=0  OutDataTypeStr=double
  Signal Override Switch 0 = Use Model 1 = Use Constant : Constant  Value=0
  Out1 : Outport
  wires:
  Override Value/1 -> Multiport Switch/3
  Multiport Switch/1 -> Out1/1
  In1/1 -> Multiport Switch/2
  Signal Override Switch 0 = Use Model 1 = Use Constant/1 -> Multiport Switch/1

== system lib_FaultDetection/Camaro Fault Detection/Input Conversions/ECM_Conversions/Override  Engine_Temp[DegC] ==
  note: This subsystem is used to override the model value of a signal to a constant value
  note: Override Switch Subsystem
  In1 : Inport
  Multiport Switch : MultiPortSwitch  DataPortOrder=Zero-based contiguous  Inputs=2  zeroidx=on
  Override Value : Constant  Value=0  OutDataTypeStr=double
  Signal Override Switch 0 = Use Model 1 = Use Constant : Constant  Value=0
  Out1 : Outport
  wires:
  Signal Override Switch 0 = Use Model 1 = Use Constant/1 -> Multiport Switch/1
  In1/1 -> Multiport Switch/2
  Multiport Switch/1 -> Out1/1
  Override Value/1 -> Multiport Switch/3

== system lib_FaultDetection/Camaro Fault Detection/Input Conversions/MCU_Conversions/Override  DC_Bus_Voltage ==
  note: This subsystem is used to override the model value of a signal to a constant value
  note: Override Switch Subsystem
  In1 : Inport
  Multiport Switch : MultiPortSwitch  DataPortOrder=Zero-based contiguous  Inputs=2  zeroidx=on
  Override Value : Constant  Value=0  OutDataTypeStr=double
  Signal Override Switch 0 = Use Model 1 = Use Constant : Constant  Value=0
  Out1 : Outport
  wires:
  Signal Override Switch 0 = Use Model 1 = Use Constant/1 -> Multiport Switch/1
  In1/1 -> Multiport Switch/2
  Multiport Switch/1 -> Out1/1
  Override Value/1 -> Multiport Switch/3

== system lib_FaultDetection/Camaro Fault Detection/Input Conversions/MCU_Conversions/Override  Direction_feedback ==
  note: This subsystem is used to override the model value of a signal to a constant value
  note: Override Switch Subsystem
  In1 : Inport
  Multiport Switch : MultiPortSwitch  DataPortOrder=Zero-based contiguous  Inputs=2  zeroidx=on
  Override Value : Constant  Value=0  OutDataTypeStr=double
  Signal Override Switch 0 = Use Model 1 = Use Constant : Constant  Value=0
  Out1 : Outport
  wires:
  Signal Override Switch 0 = Use Model 1 = Use Constant/1 -> Multiport Switch/1
  In1/1 -> Multiport Switch/2
  Multiport Switch/1 -> Out1/1
  Override Value/1 -> Multiport Switch/3

== system lib_FaultDetection/Camaro Fault Detection/Input Conversions/MCU_Conversions/Override  Inverter_enable_state ==
  note: Override Switch Subsystem
  note: This subsystem is used to override the model value of a signal to a constant value
  In1 : Inport
  Multiport Switch : MultiPortSwitch  DataPortOrder=Zero-based contiguous  Inputs=2  zeroidx=on
  Override Value : Constant  Value=0  OutDataTypeStr=double
  Signal Override Switch 0 = Use Model 1 = Use Constant : Constant  Value=0
  Out1 : Outport
  wires:
  Override Value/1 -> Multiport Switch/3
  Multiport Switch/1 -> Out1/1
  In1/1 -> Multiport Switch/2
  Signal Override Switch 0 = Use Model 1 = Use Constant/1 -> Multiport Switch/1

== system lib_FaultDetection/Camaro Fault Detection/Input Conversions/MCU_Conversions/Override  Motor_Direction ==
  note: Override Switch Subsystem
  note: This subsystem is used to override the model value of a signal to a constant value
  In1 : Inport
  Multiport Switch : MultiPortSwitch  DataPortOrder=Zero-based contiguous  Inputs=2  zeroidx=on
  Override Value : Constant  Value=0  OutDataTypeStr=double
  Signal Override Switch 0 = Use Model 1 = Use Constant : Constant  Value=0
  Out1 : Outport
  wires:
  Override Value/1 -> Multiport Switch/3
  Multiport Switch/1 -> Out1/1
  In1/1 -> Multiport Switch/2
  Signal Override Switch 0 = Use Model 1 = Use Constant/1 -> Multiport Switch/1

== system lib_FaultDetection/Camaro Fault Detection/Input Conversions/MCU_Conversions/Override  Torq_Feedback ==
  note: Override Switch Subsystem
  note: This subsystem is used to override the model value of a signal to a constant value
  In1 : Inport
  Multiport Switch : MultiPortSwitch  DataPortOrder=Zero-based contiguous  Inputs=2  zeroidx=on
  Override Value : Constant  Value=0  OutDataTypeStr=double
  Signal Override Switch 0 = Use Model 1 = Use Constant : Constant  Value=0
  Out1 : Outport
  wires:
  Override Value/1 -> Multiport Switch/3
  Multiport Switch/1 -> Out1/1
  In1/1 -> Multiport Switch/2
  Signal Override Switch 0 = Use Model 1 = Use Constant/1 -> Multiport Switch/1

== system lib_FaultDetection/Camaro Fault Detection/Input Conversions/MCU_Conversions/Override  rollingAliveCnt [123] ==
  note: Override Switch Subsystem
  note: This subsystem is used to override the model value of a signal to a constant value
  In1 : Inport
  Multiport Switch : MultiPortSwitch  DataPortOrder=Zero-based contiguous  Inputs=2  zeroidx=on
  Override Value : Constant  Value=0  OutDataTypeStr=double
  Signal Override Switch 0 = Use Model 1 = Use Constant : Constant  Value=0
  Out1 : Outport
  wires:
  Override Value/1 -> Multiport Switch/3
  Multiport Switch/1 -> Out1/1
  In1/1 -> Multiport Switch/2
  Signal Override Switch 0 = Use Model 1 = Use Constant/1 -> Multiport Switch/1
